simulink model "week1_que1"  (R2020b)
settings: Solver=VariableStepAuto  StartTime=0.0  StopTime=10.0  RelTol=1e-3
model workspace (MAT data in the model file):
  a = Simulink.Parameter
  a.Value = 2
  a.DataType = 'auto'
  a.Dimensions = [1 1]
  b = Simulink.Parameter
  b.Value = 50
  b.DataType = 'auto'
  b.Dimensions = [1 1]
  k1 = Simulink.Parameter
  k1.Value = 50
  k1.DataType = 'auto'
  k1.Dimensions = [1 1]
  m1 = Simulink.Parameter
  m1.Value = 100
  m1.DataType = 'auto'
  m1.Dimensions = [1 1]
  m2 = Simulink.Parameter
  m2.Value = 25
  m2.DataType = 'auto'
  m2.Dimensions = [1 1]
  w = Simulink.Parameter
  w.Value = 10
  w.DataType = 'auto'
  w.Dimensions = [1 1]
values from neighbouring files (symbols this model uses):
  a = 2    [Que1.mat]
  b = 50    [Que1.mat]
  k1 = 50    [Que1.mat]
  m1 = 100    [Que1.mat]
  m2 = 25.31    [Que1.mat]
  w = 10    [Que1.mat]
settings Model: Creator=hp  LastModifiedBy=hp

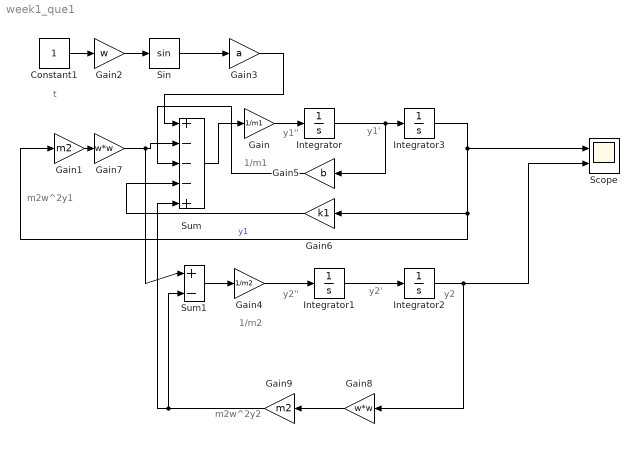
== system week1_que1 ==
  note: 1/m2
  note: y1''
  note: y1'
  note: y2'
  note: m2w^2y1
  note: t
  note: 1/m1
  note: m2w^2y2
  note: y2
  note: y2''
  Constant1 : Constant
  Gain : Gain  Gain=1/m1
  Gain1 : Gain  Gain=m2
  Gain2 : Gain  Gain=w
  Gain3 : Gain  Gain=a
  Gain4 : Gain  Gain=1/m2
  Gain5 : Gain  Gain=b
  Gain6 : Gain  Gain=k1
  Gain7 : Gain  Gain=w*w
  Gain8 : Gain  Gain=w*w
  Gain9 : Gain  Gain=m2
  Integrator{,1..3} (4 alike) : Integrator
  Scope : Scope  NumInputPorts=2
  Sin : Trigonometry
  Sum : Sum  Inputs=+---+
  Sum1 : Sum  Inputs=|+-
  wires:
  Gain4/1 -> Integrator1/1
  Sum/1 -> Gain/1
  Integrator1/1 -> Integrator2/1
  Gain7/1 -> Sum1/1, Sum/2
  Gain2/1 -> Sin/1
  Constant1/1 -> Gain2/1
  Gain8/1 -> Gain9/1
  Integrator/1 -> Gain5/1, Integrator3/1
  Gain5/1 -> Sum/3
  Gain1/1 -> Gain7/1
  Sum1/1 -> Gain4/1
  Gain6/1 -> Sum/4
  Gain3/1 -> Sum/1
  Integrator3/1 -> Gain6/1, Gain1/1, Scope/1  "y1"
  Gain9/1 -> Sum1/2, Sum/5
  Integrator2/1 -> Gain8/1, Scope/2
  Sin/1 -> Gain3/1
  Gain/1 -> Integrator/1
